simulink model "universalshiftregister"  (R2023a)
settings: Solver=VariableStepAuto  StartTime=0.0  StopTime=10.0  RelTol=1e-3
libraries: simulink_extras x4
settings Model: Creator=prath  LastModifiedBy=prath

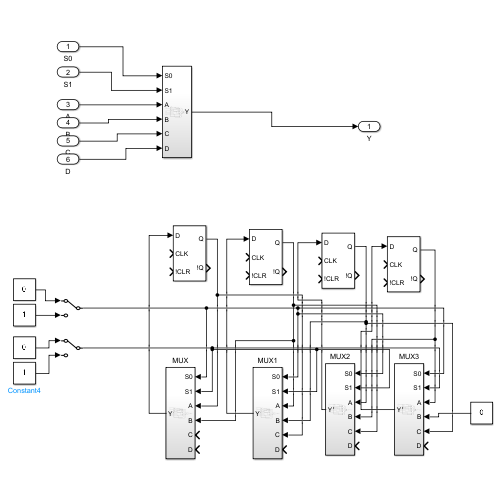
[thumbnail: Simulink's stored preview of the top-level diagram]
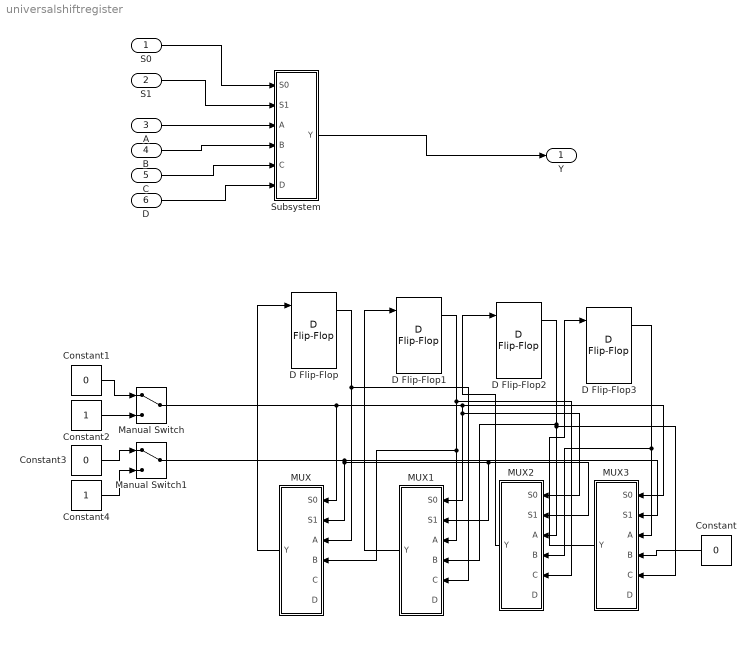
== system universalshiftregister ==
  S0 : Inport
  S1 : Inport  Port=2
  A : Inport  Port=3
  B : Inport  Port=4
  C : Inport  Port=5
  D : Inport  Port=6
  Constant : Constant  Value=0
  Constant1 : Constant  Value=0
  Constant2 : Constant
  Constant3 : Constant  Value=0
  Constant4 : Constant
  D Flip-Flop{,1..3} (4 alike) : simulink_extras/Flip Flops/D Flip-Flop
  MUX : Subsystem
  MUX1 : Subsystem
  MUX2 : Subsystem
  MUX3 : Subsystem
  Manual Switch : ManualSwitch
  Manual Switch1 : ManualSwitch
  Subsystem : Subsystem
  Y : Outport
  wires:
  S0/1 -> Subsystem/1(S0)
  S1/1 -> Subsystem/2(S1)
  A/1 -> Subsystem/3(A)
  B/1 -> Subsystem/4(B)
  C/1 -> Subsystem/5(C)
  D/1 -> Subsystem/6(D)
  Subsystem/1(Y) -> Y/1
  D Flip-Flop2/1 -> MUX3/5(C), MUX2/3(A), MUX1/4(B)
  D Flip-Flop1/1 -> MUX2/5(C), MUX/4(B), MUX1/3(A)
  D Flip-Flop/1 -> MUX1/5(C), MUX/3(A)
  D Flip-Flop3/1 -> MUX2/4(B), MUX3/3(A)
  Constant/1 -> MUX3/4(B)
  Constant1/1 -> Manual Switch/1
  Constant2/1 -> Manual Switch/2
  Constant3/1 -> Manual Switch1/1
  Constant4/1 -> Manual Switch1/2
  Manual Switch/1 -> MUX3/1(S0), MUX2/1(S0), MUX1/1(S0), MUX/1(S0)
  Manual Switch1/1 -> MUX3/2(S1), MUX2/2(S1), MUX1/2(S1), MUX/2(S1)
  MUX/1(Y) -> D Flip-Flop/1
  MUX1/1(Y) -> D Flip-Flop1/1
  MUX2/1(Y) -> D Flip-Flop2/1
  MUX3/1(Y) -> D Flip-Flop3/1

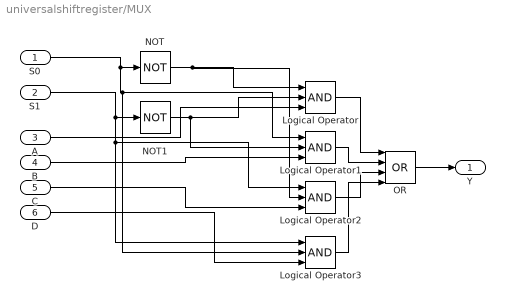
== system universalshiftregister/MUX ==
  S0 : Inport
  S1 : Inport  Port=2
  A : Inport  Port=3
  B : Inport  Port=4
  C : Inport  Port=5
  D : Inport  Port=6
  Logical Operator{,1..3} (4 alike) : Logic  Inputs=3  AllPortsSameDT=off  OutDataTypeStr=boolean
  NOT : Logic  Operator=NOT  IconShape=distinctive  AllPortsSameDT=off  OutDataTypeStr=boolean
  NOT1 : Logic  Operator=NOT  IconShape=distinctive  AllPortsSameDT=off  OutDataTypeStr=boolean
  OR : Logic  Operator=OR  Inputs=4  IconShape=distinctive  AllPortsSameDT=off  OutDataTypeStr=boolean
  Y : Outport
  wires:
  NOT1/1 -> Logical Operator1/2, Logical Operator/2
  C/1 -> Logical Operator2/3
  D/1 -> Logical Operator3/3
  NOT/1 -> Logical Operator2/2, Logical Operator/1
  S1/1 -> Logical Operator3/1, Logical Operator2/1, NOT1/1
  OR/1 -> Y/1
  S0/1 -> Logical Operator3/2, Logical Operator1/1, NOT/1
  A/1 -> Logical Operator/3
  B/1 -> Logical Operator1/3
  Logical Operator1/1 -> OR/2
  Logical Operator3/1 -> OR/4
  Logical Operator2/1 -> OR/3
  Logical Operator/1 -> OR/1

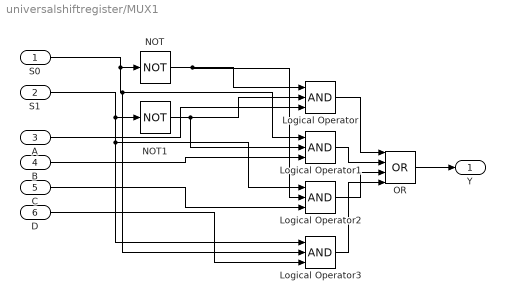
== system universalshiftregister/MUX1 ==
  S0 : Inport
  S1 : Inport  Port=2
  A : Inport  Port=3
  B : Inport  Port=4
  C : Inport  Port=5
  D : Inport  Port=6
  Logical Operator{,1..3} (4 alike) : Logic  Inputs=3  AllPortsSameDT=off  OutDataTypeStr=boolean
  NOT : Logic  Operator=NOT  IconShape=distinctive  AllPortsSameDT=off  OutDataTypeStr=boolean
  NOT1 : Logic  Operator=NOT  IconShape=distinctive  AllPortsSameDT=off  OutDataTypeStr=boolean
  OR : Logic  Operator=OR  Inputs=4  IconShape=distinctive  AllPortsSameDT=off  OutDataTypeStr=boolean
  Y : Outport
  wires:
  NOT1/1 -> Logical Operator1/2, Logical Operator/2
  C/1 -> Logical Operator2/3
  D/1 -> Logical Operator3/3
  NOT/1 -> Logical Operator2/2, Logical Operator/1
  S1/1 -> Logical Operator3/1, Logical Operator2/1, NOT1/1
  OR/1 -> Y/1
  S0/1 -> Logical Operator3/2, Logical Operator1/1, NOT/1
  A/1 -> Logical Operator/3
  B/1 -> Logical Operator1/3
  Logical Operator1/1 -> OR/2
  Logical Operator3/1 -> OR/4
  Logical Operator2/1 -> OR/3
  Logical Operator/1 -> OR/1

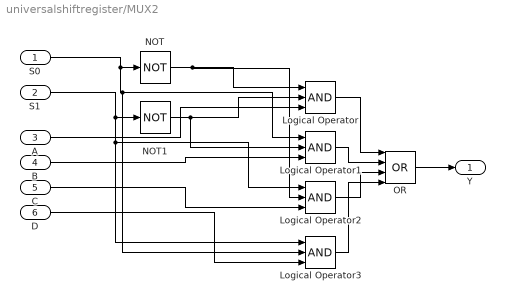
== system universalshiftregister/MUX2 ==
  S0 : Inport
  S1 : Inport  Port=2
  A : Inport  Port=3
  B : Inport  Port=4
  C : Inport  Port=5
  D : Inport  Port=6
  Logical Operator{,1..3} (4 alike) : Logic  Inputs=3  AllPortsSameDT=off  OutDataTypeStr=boolean
  NOT : Logic  Operator=NOT  IconShape=distinctive  AllPortsSameDT=off  OutDataTypeStr=boolean
  NOT1 : Logic  Operator=NOT  IconShape=distinctive  AllPortsSameDT=off  OutDataTypeStr=boolean
  OR : Logic  Operator=OR  Inputs=4  IconShape=distinctive  AllPortsSameDT=off  OutDataTypeStr=boolean
  Y : Outport
  wires:
  NOT1/1 -> Logical Operator1/2, Logical Operator/2
  C/1 -> Logical Operator2/3
  D/1 -> Logical Operator3/3
  NOT/1 -> Logical Operator2/2, Logical Operator/1
  S1/1 -> Logical Operator3/1, Logical Operator2/1, NOT1/1
  OR/1 -> Y/1
  S0/1 -> Logical Operator3/2, Logical Operator1/1, NOT/1
  A/1 -> Logical Operator/3
  B/1 -> Logical Operator1/3
  Logical Operator1/1 -> OR/2
  Logical Operator3/1 -> OR/4
  Logical Operator2/1 -> OR/3
  Logical Operator/1 -> OR/1

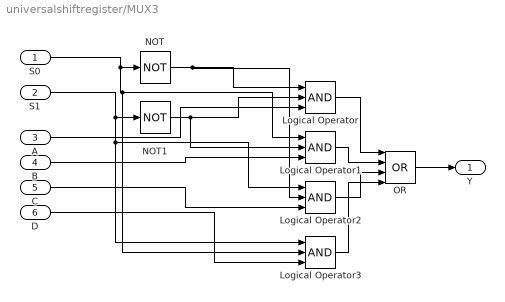
== system universalshiftregister/MUX3 ==
  S0 : Inport
  S1 : Inport  Port=2
  A : Inport  Port=3
  B : Inport  Port=4
  C : Inport  Port=5
  D : Inport  Port=6
  Logical Operator{,1..3} (4 alike) : Logic  Inputs=3  AllPortsSameDT=off  OutDataTypeStr=boolean
  NOT : Logic  Operator=NOT  IconShape=distinctive  AllPortsSameDT=off  OutDataTypeStr=boolean
  NOT1 : Logic  Operator=NOT  IconShape=distinctive  AllPortsSameDT=off  OutDataTypeStr=boolean
  OR : Logic  Operator=OR  Inputs=4  IconShape=distinctive  AllPortsSameDT=off  OutDataTypeStr=boolean
  Y : Outport
  wires:
  NOT1/1 -> Logical Operator1/2, Logical Operator/2
  C/1 -> Logical Operator2/3
  D/1 -> Logical Operator3/3
  NOT/1 -> Logical Operator2/2, Logical Operator/1
  S1/1 -> Logical Operator3/1, Logical Operator2/1, NOT1/1
  OR/1 -> Y/1
  S0/1 -> Logical Operator3/2, Logical Operator1/1, NOT/1
  A/1 -> Logical Operator/3
  B/1 -> Logical Operator1/3
  Logical Operator1/1 -> OR/2
  Logical Operator3/1 -> OR/4
  Logical Operator2/1 -> OR/3
  Logical Operator/1 -> OR/1

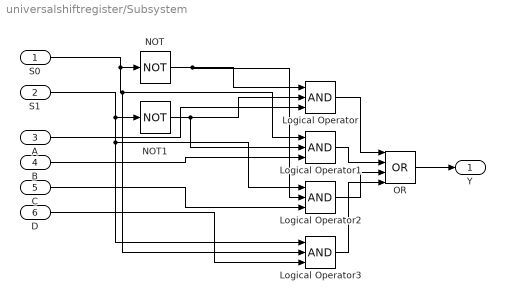
== system universalshiftregister/Subsystem ==
  S0 : Inport
  S1 : Inport  Port=2
  A : Inport  Port=3
  B : Inport  Port=4
  C : Inport  Port=5
  D : Inport  Port=6
  Logical Operator{,1..3} (4 alike) : Logic  Inputs=3  AllPortsSameDT=off  OutDataTypeStr=boolean
  NOT : Logic  Operator=NOT  IconShape=distinctive  AllPortsSameDT=off  OutDataTypeStr=boolean
  NOT1 : Logic  Operator=NOT  IconShape=distinctive  AllPortsSameDT=off  OutDataTypeStr=boolean
  OR : Logic  Operator=OR  Inputs=4  IconShape=distinctive  AllPortsSameDT=off  OutDataTypeStr=boolean
  Y : Outport
  wires:
  NOT1/1 -> Logical Operator1/2, Logical Operator/2
  C/1 -> Logical Operator2/3
  D/1 -> Logical Operator3/3
  NOT/1 -> Logical Operator2/2, Logical Operator/1
  S1/1 -> Logical Operator3/1, Logical Operator2/1, NOT1/1
  OR/1 -> Y/1
  S0/1 -> Logical Operator3/2, Logical Operator1/1, NOT/1
  A/1 -> Logical Operator/3
  B/1 -> Logical Operator1/3
  Logical Operator1/1 -> OR/2
  Logical Operator3/1 -> OR/4
  Logical Operator2/1 -> OR/3
  Logical Operator/1 -> OR/1
